simulink model "ex5"  (Simulink 6.0)
settings: Solver=VariableStepDiscrete  StartTime=0.0  StopTime=100000  RelTol=1e-3
libraries: commchan2 x1, commsink2 x1, dspmathops x1, commrandsrc2 x1
settings Model: LastModifiedBy=lxy

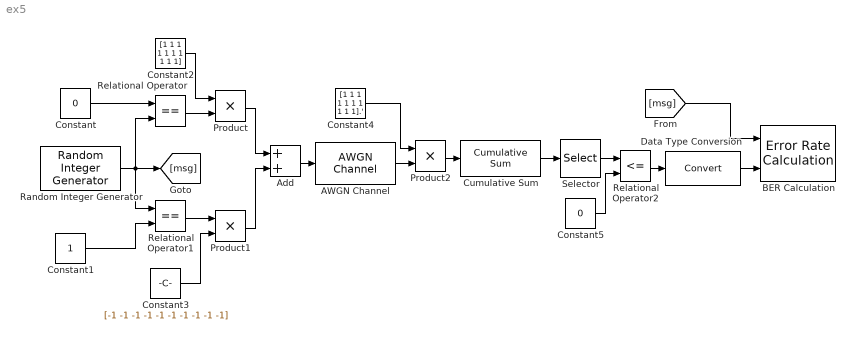
== system ex5 ==
  AWGN Channel : commchan2/AWGN Channel  seed=67  noiseMode="Signal to noise ratio  (Eb/No)"  EbNodB=SNR  EsNodB=10  SNRdB=-7  bitsPerSym=1  Ps=1  Tsym=1  variance=1
  Add : Sum  OutScaling=2^-10
  BER Calculation : commsink2/Error Rate Calculation  N=0  st_delay=0  cp_mode=Entire frame  subframe=[]  PMode=Workspace  WsName=BER  RsMode2=off  stop=off  numErr=100  maxBits=1e6
  Constant : Constant  Value=0
  Constant1 : Constant
  Constant2 : Constant  Value=[1 1 1 1 1 1 1 1 1 1]  SampleTime=0.1
  Constant3 : Constant  Value=[-1 -1 -1 -1 -1 -1 -1 -1 -1 -1]  SampleTime=0.1
  Constant4 : Constant  Value=[1 1 1 1 1 1 1 1 1 1].'
  Constant5 : Constant  Value=0
  Cumulative Sum : dspmathops/Cumulative Sum  DialogController=dspDDGCreate  DialogControllerArgs=DataTag0  dim=Rows  reset_popup=None  roundingMode=Floor  overflowMode=off
  Data Type Conversion : DataTypeConversion  OutDataTypeMode=double
  Product : Product  RndMeth=Zero
  Product1 : Product  RndMeth=Zero
  Product2 : Product  RndMeth=Zero
  Random Integer Generator : commrandsrc2/Random Integer Generator  mul=2  seed=1234  Ts=1  frameBased=off  sampPerFrame=1  orient=off
  Relational Operator : RelationalOperator  Operator===  LogicOutDataTypeMode=Boolean
  Relational Operator1 : RelationalOperator  Operator===  LogicOutDataTypeMode=Boolean
  Relational Operator2 : RelationalOperator  Operator=<=  LogicOutDataTypeMode=Boolean
  Selector : Selector  Elements=[10]  InputPortWidth=10
  wires:
  Constant/1 -> Relational Operator/1
  Constant1/1 -> Relational Operator1/2
  Relational Operator1/1 -> Product1/1
  Constant3/1 -> Product1/2
  Product1/1 -> Add/2
  Product/1 -> Add/1
  Add/1 -> AWGN Channel/1
  Constant4/1 -> Product2/1
  AWGN Channel/1 -> Product2/2
  Product2/1 -> Cumulative Sum/1
  Cumulative Sum/1 -> Selector/1
  Selector/1 -> Relational Operator2/1
  Relational Operator2/1 -> Data Type Conversion/1
  Random Integer Generator/1 -> Relational Operator1/1, Relational Operator/2, [msg]
  Relational Operator/1 -> Product/2
  Constant2/1 -> Product/1
  [msg] -> BER Calculation/1
  Data Type Conversion/1 -> BER Calculation/2
  Constant5/1 -> Relational Operator2/2
